simulink model "asbdhc2"  (Simulink 8.0)
settings: Solver=ode45  StartTime=0.0  StopTime=1000  MaxStep=1/30  RelTol=1e-2  AbsTol=1e-3
PreLoadFcn:
  | load asbdhc2_init;
values from neighbouring files (symbols this model uses):
  beaver_b = 14.63    [beaver_4_14_2013.mat]    (also in modelScript.m = 1.4224; monteCarloSim01.mat = 1.4224; simData_12_10_2013.mat = 1.4224; simData_12_9_2013.mat = 1.4224)
  beaver_c = 1.5875    [beaver_4_14_2013.mat]    (also in modelScript.m = 0.3302; monteCarloSim01.mat = 0.3302; simData_12_10_2013.mat = 0.3302; simData_12_9_2013.mat = 0.3302)
  beaver_init_p = 0    [beaver_4_14_2013.mat]    (also in monteCarloSim01.mat; simData_12_10_2013.mat; simData_12_9_2013.mat; simData_4_23_2013.mat)
  beaver_init_pitch = 0.13029612885    [beaver_4_14_2013.mat]    (also in monteCarloSim01.mat; simData_12_10_2013.mat; simData_12_9_2013.mat; simData_4_23_2013.mat)
  beaver_init_q = 0    [beaver_4_14_2013.mat]    (also in monteCarloSim01.mat; simData_12_10_2013.mat; simData_12_9_2013.mat; simData_4_23_2013.mat)
  beaver_init_r = 0    [beaver_4_14_2013.mat]    (also in monteCarloSim01.mat; simData_12_10_2013.mat; simData_12_9_2013.mat; simData_4_23_2013.mat)
  beaver_init_roll = 0    [beaver_4_14_2013.mat]    (also in monteCarloSim01.mat; simData_12_10_2013.mat; simData_12_9_2013.mat; simData_4_23_2013.mat)
  beaver_mass = 2288.231    [beaver_4_14_2013.mat]    (also in modelScript.m = 1.56; monteCarloSim01.mat = 1.56; simData_12_10_2013.mat = 1.56; simData_12_9_2013.mat = 1.56)
  beaver_S = 23.23    [beaver_4_14_2013.mat]    (also in modelScript.m = 0.2589; monteCarloSim01.mat = 0.2589; simData_12_10_2013.mat = 0.2589; simData_12_9_2013.mat = 0.2589)
  CD0 = 0.03    [modelScript.m]    (also in monteCarloSim01.mat; polarFun.m = x(1); simData_12_10_2013.mat; simData_12_9_2013.mat)
  Cl0 = 0.000591    [beaver_4_14_2013.mat]    (also in monteCarloSim01.mat; simData_12_10_2013.mat; simData_12_9_2013.mat; simData_4_23_2013.mat)
  Cl_alpha2_dpt = -0.01406    [beaver_4_14_2013.mat]    (also in monteCarloSim01.mat; simData_12_10_2013.mat; simData_12_9_2013.mat; simData_4_23_2013.mat)
  Cl_beta = -0.0618    [beaver_4_14_2013.mat]    (also in monteCarloSim01.mat; simData_12_10_2013.mat; simData_12_9_2013.mat; simData_4_23_2013.mat)
  Cl_da = -0.09917    [beaver_4_14_2013.mat]    (also in monteCarloSim01.mat; simData_12_10_2013.mat; simData_12_9_2013.mat; simData_4_23_2013.mat)
  Cl_da_alpha = -0.08269    [beaver_4_14_2013.mat]    (also in monteCarloSim01.mat; simData_12_10_2013.mat; simData_12_9_2013.mat; simData_4_23_2013.mat)
  Cl_dr = 0.006934    [beaver_4_14_2013.mat]    (also in monteCarloSim01.mat; simData_12_10_2013.mat; simData_12_9_2013.mat; simData_4_23_2013.mat)
  Cl_p = -0.5045    [beaver_4_14_2013.mat]    (also in monteCarloSim01.mat; simData_12_10_2013.mat; simData_12_9_2013.mat; simData_4_23_2013.mat)
  Cl_r = 0.1695    [beaver_4_14_2013.mat]    (also in monteCarloSim01.mat; simData_12_10_2013.mat; simData_12_9_2013.mat; simData_4_23_2013.mat)
  Cm0 = 0.09448    [beaver_4_14_2013.mat]    (also in monteCarloSim01.mat; simData_12_10_2013.mat; simData_12_9_2013.mat; simData_4_23_2013.mat)
  Cm_alpha = -0.6028    [beaver_4_14_2013.mat]    (also in monteCarloSim01.mat; simData_12_10_2013.mat; simData_12_9_2013.mat; simData_4_23_2013.mat)
  Cm_alpha2 = -2.14    [beaver_4_14_2013.mat]    (also in monteCarloSim01.mat; simData_12_10_2013.mat; simData_12_9_2013.mat; simData_4_23_2013.mat)
  Cm_beta2 = 0.6921    [beaver_4_14_2013.mat]    (also in monteCarloSim01.mat; simData_12_10_2013.mat; simData_12_9_2013.mat; simData_4_23_2013.mat)
  Cm_de = -1.921    [beaver_4_14_2013.mat]    (also in monteCarloSim01.mat; simData_12_10_2013.mat; simData_12_9_2013.mat; simData_4_23_2013.mat)
  Cm_df = 0.4072    [beaver_4_14_2013.mat]    (also in monteCarloSim01.mat; simData_12_10_2013.mat; simData_12_9_2013.mat; simData_4_23_2013.mat)
  Cm_dpt = -0.07895    [beaver_4_14_2013.mat]    (also in monteCarloSim01.mat; simData_12_10_2013.mat; simData_12_9_2013.mat; simData_4_23_2013.mat)
  Cm_q = -15.56    [beaver_4_14_2013.mat]    (also in monteCarloSim01.mat; simData_12_10_2013.mat; simData_12_9_2013.mat; simData_4_23_2013.mat)
  Cm_r = -0.3118    [beaver_4_14_2013.mat]    (also in monteCarloSim01.mat; simData_12_10_2013.mat; simData_12_9_2013.mat; simData_4_23_2013.mat)
  Cn0 = -0.003117    [beaver_4_14_2013.mat]    (also in monteCarloSim01.mat; simData_12_10_2013.mat; simData_12_9_2013.mat; simData_4_23_2013.mat)
  Cn_beta = 0.006719    [beaver_4_14_2013.mat]    (also in monteCarloSim01.mat; simData_12_10_2013.mat; simData_12_9_2013.mat; simData_4_23_2013.mat)
  Cn_beta3 = 0.1373    [beaver_4_14_2013.mat]    (also in monteCarloSim01.mat; simData_12_10_2013.mat; simData_12_9_2013.mat; simData_4_23_2013.mat)
  Cn_da = -0.003872    [beaver_4_14_2013.mat]    (also in monteCarloSim01.mat; simData_12_10_2013.mat; simData_12_9_2013.mat; simData_4_23_2013.mat)
  Cn_dpt3 = -0.003026    [beaver_4_14_2013.mat]    (also in monteCarloSim01.mat; simData_12_10_2013.mat; simData_12_9_2013.mat; simData_4_23_2013.mat)
  Cn_dr = -0.08265    [beaver_4_14_2013.mat]    (also in monteCarloSim01.mat; simData_12_10_2013.mat; simData_12_9_2013.mat; simData_4_23_2013.mat)
  Cn_p = -0.1585    [beaver_4_14_2013.mat]    (also in monteCarloSim01.mat; simData_12_10_2013.mat; simData_12_9_2013.mat; simData_4_23_2013.mat)
  Cn_q = 0.1595    [beaver_4_14_2013.mat]    (also in monteCarloSim01.mat; simData_12_10_2013.mat; simData_12_9_2013.mat; simData_4_23_2013.mat)
  Cn_r = -0.1112    [beaver_4_14_2013.mat]    (also in monteCarloSim01.mat; simData_12_10_2013.mat; simData_12_9_2013.mat; simData_4_23_2013.mat)
  Cx0 = -0.03554    [beaver_4_14_2013.mat]    (also in modelScript.m = 0; monteCarloSim01.mat = 0; simData_12_10_2013.mat = 0; simData_12_9_2013.mat = 0)
  Cx_alpha = 0.00292    [beaver_4_14_2013.mat]    (also in modelScript.m = 0; monteCarloSim01.mat = 0; simData_12_10_2013.mat = 0; simData_12_9_2013.mat = 0)
  Cx_alpha2 = 5.459    [beaver_4_14_2013.mat]    (also in modelScript.m = 0; monteCarloSim01.mat = 0; simData_12_10_2013.mat = 0; simData_12_9_2013.mat = 0)
  Cx_alpha3 = -5.162    [beaver_4_14_2013.mat]    (also in modelScript.m = 0; monteCarloSim01.mat = 0; simData_12_10_2013.mat = 0; simData_12_9_2013.mat = 0)
  Cx_df = -0.09447    [beaver_4_14_2013.mat]    (also in modelScript.m = 0; monteCarloSim01.mat = 0; simData_12_10_2013.mat = 0; simData_12_9_2013.mat = 0)
  Cx_df_alpha = 1.106    [beaver_4_14_2013.mat]    (also in modelScript.m = 0; monteCarloSim01.mat = 0; simData_12_10_2013.mat = 0; simData_12_9_2013.mat = 0)
  Cx_dpt = 0.1161    [beaver_4_14_2013.mat]    (also in modelScript.m = 0; monteCarloSim01.mat = 0; simData_12_10_2013.mat = 0; simData_12_9_2013.mat = 0)
  Cx_dpt2_alpha = 0.1453    [beaver_4_14_2013.mat]    (also in modelScript.m = 0; monteCarloSim01.mat = 0; simData_12_10_2013.mat = 0; simData_12_9_2013.mat = 0)
  Cx_dr = 0.03412    [beaver_4_14_2013.mat]    (also in modelScript.m = 0; monteCarloSim01.mat = 0; simData_12_10_2013.mat = 0; simData_12_9_2013.mat = 0)
  Cx_q = -0.6748    [beaver_4_14_2013.mat]    (also in modelScript.m = 0; monteCarloSim01.mat = 0; simData_12_10_2013.mat = 0; simData_12_9_2013.mat = 0)
  Cy0 = -0.002226    [beaver_4_14_2013.mat]    (also in modelScript.m = 0; monteCarloSim01.mat = 0; simData_12_10_2013.mat = 0; simData_12_9_2013.mat = 0)
  Cy_beta = -0.7678    [beaver_4_14_2013.mat]    (also in modelScript.m = 0; monteCarloSim01.mat = 0; simData_12_10_2013.mat = 0; simData_12_9_2013.mat = 0)
  Cy_da = -0.02956    [beaver_4_14_2013.mat]    (also in modelScript.m = 0; monteCarloSim01.mat = 0; simData_12_10_2013.mat = 0; simData_12_9_2013.mat = 0)
  Cy_dr = 0.1158    [beaver_4_14_2013.mat]    (also in modelScript.m = 0; monteCarloSim01.mat = 0; simData_12_10_2013.mat = 0; simData_12_9_2013.mat = 0)
  Cy_dr_alpha = 0.5238    [beaver_4_14_2013.mat]    (also in modelScript.m = 0; monteCarloSim01.mat = 0; simData_12_10_2013.mat = 0; simData_12_9_2013.mat = 0)
  Cy_p = -0.124    [beaver_4_14_2013.mat]    (also in modelScript.m = 0; monteCarloSim01.mat = 0; simData_12_10_2013.mat = 0; simData_12_9_2013.mat = 0)
  Cy_r = 0.3666    [beaver_4_14_2013.mat]    (also in modelScript.m = 0; monteCarloSim01.mat = 0; simData_12_10_2013.mat = 0; simData_12_9_2013.mat = 0)
  Cz0 = -0.05504    [beaver_4_14_2013.mat]    (also in modelScript.m = 0; monteCarloSim01.mat = 0; simData_12_10_2013.mat = 0; simData_12_9_2013.mat = 0)
  Cz_alpha = -5.578    [beaver_4_14_2013.mat]    (also in modelScript.m = 0; monteCarloSim01.mat = 0; simData_12_10_2013.mat = 0; simData_12_9_2013.mat = 0)
  Cz_alpha3 = 3.442    [beaver_4_14_2013.mat]    (also in modelScript.m = 0; monteCarloSim01.mat = 0; simData_12_10_2013.mat = 0; simData_12_9_2013.mat = 0)
  Cz_de = -0.398    [beaver_4_14_2013.mat]    (also in modelScript.m = 0; monteCarloSim01.mat = 0; simData_12_10_2013.mat = 0; simData_12_9_2013.mat = 0)
  Cz_de_beta = -15.93    [beaver_4_14_2013.mat]    (also in modelScript.m = 0; monteCarloSim01.mat = 0; simData_12_10_2013.mat = 0; simData_12_9_2013.mat = 0)
  Cz_df = -1.377    [beaver_4_14_2013.mat]    (also in modelScript.m = 0; monteCarloSim01.mat = 0; simData_12_10_2013.mat = 0; simData_12_9_2013.mat = 0)
  Cz_df_alpha = -1.261    [beaver_4_14_2013.mat]    (also in modelScript.m = 0; monteCarloSim01.mat = 0; simData_12_10_2013.mat = 0; simData_12_9_2013.mat = 0)
  Cz_dpt = -0.1563    [beaver_4_14_2013.mat]    (also in modelScript.m = 0; monteCarloSim01.mat = 0; simData_12_10_2013.mat = 0; simData_12_9_2013.mat = 0)
  Cz_q = -2.988    [beaver_4_14_2013.mat]    (also in modelScript.m = 0; monteCarloSim01.mat = 0; simData_12_10_2013.mat = 0; simData_12_9_2013.mat = 0)
  Ix = .1147    (= 0.1147)    [modelScript.m]    (also in monteCarloSim01.mat; simData_12_10_2013.mat; simData_12_9_2013.mat; simData_4_26_2013.mat)
  Ixz = .0015    (= 0.0015)    [modelScript.m]    (also in monteCarloSim01.mat; simData_12_10_2013.mat; simData_12_9_2013.mat; simData_4_26_2013.mat)
  Iy = .0576    (= 0.0576)    [modelScript.m]    (also in monteCarloSim01.mat; simData_12_10_2013.mat; simData_12_9_2013.mat; simData_4_26_2013.mat)
  Iz = .1712    (= 0.1712)    [modelScript.m]    (also in monteCarloSim01.mat; simData_12_10_2013.mat; simData_12_9_2013.mat; simData_4_26_2013.mat)
  KCL2 = 1/(pi*.7*beaver_b/beaver_c)    [modelScript.m]    (also in monteCarloSim01.mat = 0.0493425392361; polarFun.m = x(2); simData_12_10_2013.mat = 0.0493425392361; simData_12_9_2013.mat = 0.0493425392361)
  m = state.W/g(1)    [plant.m]
  nonLinearCd = [0.025 0.0283582705905 0.0317165411809 0.0350748117714 0.0384330823618 0.0417913529523 0.0451496235427 0.0485078941332 0.0518661647236 0.0552244353141 0.0585827059046 0.061940976495 ... (1000 elements, 1x1000)]    [NACA0012Adam.mat]    (also in monteCarloSim01.mat; simData_12_10_2013.mat; simData_12_9_2013.mat; simData_4_23_2013.mat)
  nonLinearCl = [0 0.0485067508622 0.0970135017244 0.145520252587 0.194027003449 0.240505289572 0.286480266666 0.332455243759 0.378430220853 0.421875006681 0.463843622747 0.505812238814 ... (1000 elements, 1x1000)]    [NACA0012Adam.mat]    (also in monteCarloSim01.mat; simData_12_10_2013.mat; simData_12_9_2013.mat; simData_4_23_2013.mat)
  nonLinearWindAeroAlpha = [-3.14159265359 -3.13530317881 -3.12901370403 -3.12272422924 -3.11643475446 -3.11014527968 -3.1038558049 -3.09756633012 -3.09127685533 -3.08498738055 -3.07869790577 -3.07240843099 ... (1000 elements, 1x1000)]    [NACA0012Adam.mat]    (also in monteCarloSim01.mat; simData_12_10_2013.mat; simData_12_9_2013.mat; simData_4_23_2013.mat)
  q = state.eulerRates(:,2)    [eulerKalman.m]
  r = state.eulerRates(:,3)    [eulerKalman.m]
  sampleVec = [1/1000 0]    [modelScript.m]    (also in monteCarloSim01.mat = [0.0909090909091 0]; simData_12_10_2013.mat = [0.0909090909091 0]; simData_12_9_2013.mat = [0.001 0]; simData_4_26_2013.mat = [0.02 0])
  u0 = 100/3.28    (= 30.487804878)    [modelScript.m]    (also in monteCarloSim01.mat; simData_12_10_2013.mat; simData_12_9_2013.mat; simData_4_26_2013.mat)
  uaero0 = [-0.0317656979071 -0.0320210159663 -0.0365180369264 0]    [beaver_4_14_2013.mat]    (also in monteCarloSim01.mat; simData_12_10_2013.mat; simData_12_9_2013.mat; simData_4_23_2013.mat)
  v0 = 0    [modelScript.m]    (also in monteCarloSim01.mat; simData_12_10_2013.mat; simData_12_9_2013.mat; simData_4_26_2013.mat)
  w0 = 0    [modelScript.m]    (also in monteCarloSim01.mat; simData_12_10_2013.mat; simData_12_9_2013.mat; simData_4_26_2013.mat)
undefined symbols (not defined in the file or in its folder): Earth, F, Light, MIL, s, sigbuilder_block, WGS84
libraries: aerolibconvert2 x5, aerolibtransform2 x4, aerolibadynsys x3, aerolibasang x3, aerolibwind2 x3, aerolibfltsims x3, aerolibanimutils x2, aerolib6dof2 x1, aerolibnav x1, aerolibutil x1, aerolibatmos2 x1, aerolibgravity2 x1
(part 2 of 2)

== system asbdhc2/DeHavilland Beaver Airframe/Aircraft Dynamics/Total Forces  and Moments/Aerodynamics/Body Rate Damping ==
  V : Inport
  p,q,r : Inport  Port=2
  Demux : Demux  Outputs=3
  Product : Product  SaturateOnIntegerOverflow=on  InputSameDT=on  OutDataTypeStr=Inherit: Same as first input
  Product1 : Product  SaturateOnIntegerOverflow=on  InputSameDT=on  OutDataTypeStr=Inherit: Same as first input
  Product2 : Product  SaturateOnIntegerOverflow=on  InputSameDT=on  OutDataTypeStr=Inherit: Same as first input
  Product3 : Product  Inputs=*/  SaturateOnIntegerOverflow=on  InputSameDT=on  OutDataTypeStr=Inherit: Same as first input
  Reference Length : Gain  Gain=beaver_c  SaturateOnIntegerOverflow=on  OutDataTypeStr=Inherit: Same as input  ParamDataTypeStr=Inherit: Same as input
  Reference Span : Gain  Gain=beaver_b/2  SaturateOnIntegerOverflow=on  OutDataTypeStr=Inherit: Same as input  ParamDataTypeStr=Inherit: Same as input
  "Reference Span " : Gain  Gain=beaver_b/2  SaturateOnIntegerOverflow=on  OutDataTypeStr=Inherit: Same as input  ParamDataTypeStr=Inherit: Same as input
  Sum1 : Sum  Inputs=+++  SaturateOnIntegerOverflow=on  InputSameDT=on  OutDataTypeStr=Inherit: Same as first input
  p : Subsystem
  q : Subsystem
  r : Subsystem
  Coefficients : Outport
  wires:
  p/1(delCoeff) -> Product/1
  q/1(delCoeff) -> Product1/1
  p,q,r/1 -> Demux/1
  Demux/1 -> Product/2  "p"
  Demux/2 -> Product1/2  "q"
  Demux/3 -> Product2/2  "r"
  Sum1/1 -> Product3/1
  V/1 -> Product3/2
  Product3/1 -> Coefficients/1
  Product1/1 -> Reference Length/1
  Product2/1 -> "Reference Span "/1
  Product/1 -> Reference Span/1
  r/1(delCoeff) -> Product2/1
  Reference Length/1 -> Sum1/2
  Reference Span/1 -> Sum1/1
  "Reference Span "/1 -> Sum1/3

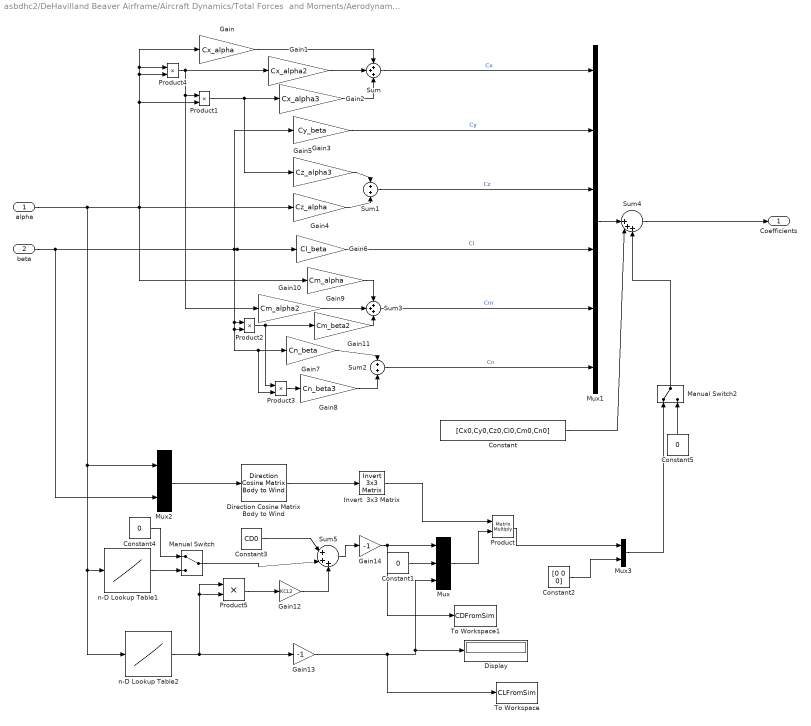
== system asbdhc2/DeHavilland Beaver Airframe/Aircraft Dynamics/Total Forces  and Moments/Aerodynamics/Datum Coefficients ==
  alpha : Inport
  beta : Inport  Port=2
  Constant : Constant  Value=[Cx0,Cy0,Cz0,Cl0,Cm0,Cn0]
  Constant1 : Constant  Value=0
  Constant2 : Constant  Value=[0 0 0]
  Constant3 : Constant  Value=CD0
  Constant4 : Constant  Value=0
  Constant5 : Constant  Value=0
  Direction Cosine Matrix Body to Wind : aerolibtransform2/Direction Cosine Matrix Body to Wind
  Display : Display
  Gain : Gain  Gain=Cx_alpha  SaturateOnIntegerOverflow=on  OutDataTypeStr=Inherit: Same as input  ParamDataTypeStr=Inherit: Same as input
  Gain1 : Gain  Gain=Cx_alpha2  SaturateOnIntegerOverflow=on  OutDataTypeStr=Inherit: Same as input  ParamDataTypeStr=Inherit: Same as input
  Gain10 : Gain  Gain=Cm_alpha2  SaturateOnIntegerOverflow=on  OutDataTypeStr=Inherit: Same as input  ParamDataTypeStr=Inherit: Same as input
  Gain11 : Gain  Gain=Cm_beta2  SaturateOnIntegerOverflow=on  OutDataTypeStr=Inherit: Same as input  ParamDataTypeStr=Inherit: Same as input
  Gain12 : Gain  Gain=KCL2
  Gain13 : Gain  Gain=-1
  Gain14 : Gain  Gain=-1
  Gain2 : Gain  Gain=Cx_alpha3  SaturateOnIntegerOverflow=on  OutDataTypeStr=Inherit: Same as input  ParamDataTypeStr=Inherit: Same as input
  Gain3 : Gain  Gain=Cy_beta  SaturateOnIntegerOverflow=on  OutDataTypeStr=Inherit: Same as input  ParamDataTypeStr=Inherit: Same as input
  Gain4 : Gain  Gain=Cz_alpha  SaturateOnIntegerOverflow=on  OutDataTypeStr=Inherit: Same as input  ParamDataTypeStr=Inherit: Same as input
  Gain5 : Gain  Gain=Cz_alpha3  SaturateOnIntegerOverflow=on  OutDataTypeStr=Inherit: Same as input  ParamDataTypeStr=Inherit: Same as input
  Gain6 : Gain  Gain=Cl_beta  SaturateOnIntegerOverflow=on  OutDataTypeStr=Inherit: Same as input  ParamDataTypeStr=Inherit: Same as input
  Gain7 : Gain  Gain=Cn_beta  SaturateOnIntegerOverflow=on  OutDataTypeStr=Inherit: Same as input  ParamDataTypeStr=Inherit: Same as input
  Gain8 : Gain  Gain=Cn_beta3  SaturateOnIntegerOverflow=on  OutDataTypeStr=Inherit: Same as input  ParamDataTypeStr=Inherit: Same as input
  Gain9 : Gain  Gain=Cm_alpha  SaturateOnIntegerOverflow=on  OutDataTypeStr=Inherit: Same as input  ParamDataTypeStr=Inherit: Same as input
  Invert  3x3 Matrix : aerolibutil/Invert  3x3 Matrix
  Manual Switch : ManualSwitch
  Manual Switch2 : ManualSwitch
  Mux : Mux  Inputs=3
  Mux1 : Mux  Inputs=6
  Mux2 : Mux  Inputs=2
  Mux3 : Mux  Inputs=[3 3]
  Product : Product  Multiplication=Matrix(*)  RndMeth=Zero
  Product{1..4} (4 alike) : Product  SaturateOnIntegerOverflow=on  InputSameDT=on  OutDataTypeStr=Inherit: Same as first input
  Product5 : Product  RndMeth=Zero
  Sum : Sum  Inputs=+++  SaturateOnIntegerOverflow=on
  Sum1 : Sum  SaturateOnIntegerOverflow=on
  Sum2 : Sum  SaturateOnIntegerOverflow=on
  Sum3 : Sum  Inputs=+++  SaturateOnIntegerOverflow=on
  Sum4 : Sum  Inputs=||+++  SaturateOnIntegerOverflow=on
  Sum5 : Sum  Inputs=|+++  SaturateOnIntegerOverflow=on
  To Workspace : ToWorkspace  VariableName=CLFromSim  SampleTime=-1  SaveFormat=Structure
  To Workspace1 : ToWorkspace  VariableName=CDFromSim  SampleTime=-1  SaveFormat=Structure
  n-D Lookup Table1 : Lookup_n-D  NumberOfTableDimensions=1  BreakpointsForDimension1=nonLinearWindAeroAlpha  Table=nonLinearCd  RndMeth=Simplest  InputSameDT=on
  n-D Lookup Table2 : Lookup_n-D  NumberOfTableDimensions=1  BreakpointsForDimension1=nonLinearWindAeroAlpha  Table=nonLinearCl  RndMeth=Simplest  InputSameDT=on
  Coefficients : Outport
  wires:
  Constant/1 -> Sum4/2
  Sum4/1 -> Coefficients/1
  Mux1/1 -> Sum4/1
  Gain10/1 -> Sum3/2
  Product2/1 -> Product3/1, Gain11/1
  Gain11/1 -> Sum3/3
  Gain9/1 -> Sum3/1
  Sum3/1 -> Mux1/5  "Cm"
  Product3/1 -> Gain8/1
  Gain8/1 -> Sum2/2
  Gain7/1 -> Sum2/1
  Gain5/1 -> Sum1/1
  Gain4/1 -> Sum1/2
  Product1/1 -> Gain5/1, Gain2/1
  Gain2/1 -> Sum/3
  Product4/1 -> Product1/1, Gain10/1, Gain1/1
  Gain1/1 -> Sum/2
  Gain/1 -> Sum/1
  Sum2/1 -> Mux1/6  "Cn"
  Sum/1 -> Mux1/1  "Cx"
  Sum1/1 -> Mux1/3  "Cz"
  Gain3/1 -> Mux1/2  "Cy"
  Gain6/1 -> Mux1/4  "Cl"
  alpha/1 -> Product1/2, Product4/2, Product4/1, Gain/1, Gain9/1, Gain4/1, Mux2/1, n-D Lookup Table2/1, n-D Lookup Table1/1
  beta/1 -> Gain3/1, Product3/2, Gain7/1, Product2/2, Product2/1, Gain6/1, Mux2/2
  Mux2/1 -> Direction Cosine Matrix Body to Wind/1
  Direction Cosine Matrix Body to Wind/1 -> Invert  3x3 Matrix/1
  Invert  3x3 Matrix/1 -> Product/1
  Constant1/1 -> Mux/2
  Gain13/1 -> Mux/3, Display/1, To Workspace/1
  Constant2/1 -> Mux3/2
  Product/1 -> Mux3/1
  n-D Lookup Table2/1 -> Product5/2, Product5/1, Gain13/1
  Mux/1 -> Product/2
  Product5/1 -> Gain12/1
  Constant3/1 -> Sum5/1
  Gain14/1 -> Mux/1, To Workspace1/1
  Sum5/1 -> Gain14/1
  Gain12/1 -> Sum5/3
  n-D Lookup Table1/1 -> Manual Switch/2
  Constant4/1 -> Manual Switch/1
  Manual Switch/1 -> Sum5/2
  Mux3/1 -> Manual Switch2/1
  Manual Switch2/1 -> Sum4/3
  Constant5/1 -> Manual Switch2/2

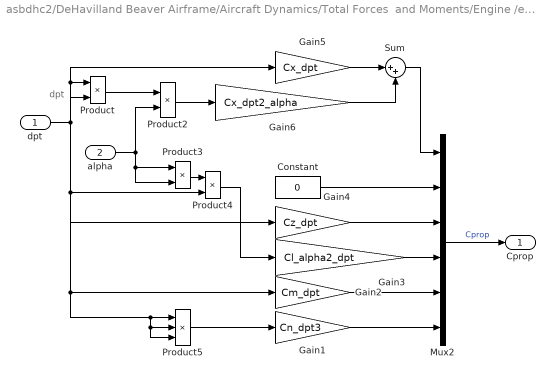
== system asbdhc2/DeHavilland Beaver Airframe/Aircraft Dynamics/Total Forces  and Moments/Engine /eng ==
  note: dpt
  dpt : Inport
  alpha : Inport  Port=2
  Constant : Constant  Value=0
  Gain1 : Gain  Gain=Cn_dpt3  SaturateOnIntegerOverflow=on  OutDataTypeStr=Inherit: Same as input  ParamDataTypeStr=Inherit: Same as input
  Gain2 : Gain  Gain=Cm_dpt  SaturateOnIntegerOverflow=on  OutDataTypeStr=Inherit: Same as input  ParamDataTypeStr=Inherit: Same as input
  Gain3 : Gain  Gain=Cl_alpha2_dpt  SaturateOnIntegerOverflow=on  OutDataTypeStr=Inherit: Same as input  ParamDataTypeStr=Inherit: Same as input
  Gain4 : Gain  Gain=Cz_dpt  SaturateOnIntegerOverflow=on  OutDataTypeStr=Inherit: Same as input  ParamDataTypeStr=Inherit: Same as input
  Gain5 : Gain  Gain=Cx_dpt  SaturateOnIntegerOverflow=on  OutDataTypeStr=Inherit: Same as input  ParamDataTypeStr=Inherit: Same as input
  Gain6 : Gain  Gain=Cx_dpt2_alpha  SaturateOnIntegerOverflow=on  OutDataTypeStr=Inherit: Same as input  ParamDataTypeStr=Inherit: Same as input
  Mux2 : Mux  Inputs=6
  Product{,2..4} (4 alike) : Product  SaturateOnIntegerOverflow=on  OutDataTypeStr=Inherit: Same as first input
  Product5 : Product  Inputs=3  SaturateOnIntegerOverflow=on  OutDataTypeStr=Inherit: Same as first input
  Sum : Sum  Inputs=|++  SaturateOnIntegerOverflow=on
  Cprop : Outport
  wires:
  Product5/1 -> Gain1/1
  Sum/1 -> Mux2/1
  Gain6/1 -> Sum/2
  Gain5/1 -> Sum/1
  Constant/1 -> Mux2/2
  Gain4/1 -> Mux2/3
  Gain3/1 -> Mux2/4
  Gain2/1 -> Mux2/5
  Gain1/1 -> Mux2/6
  Product4/1 -> Gain3/1
  Product2/1 -> Gain6/1
  dpt/1 -> Gain5/1, Product5/3, Product5/2, Product5/1, Gain2/1, Gain4/1, Product/2, Product/1, Product4/2
  alpha/1 -> Product2/2, Product3/1, Product3/2
  Mux2/1 -> Cprop/1  "Cprop"
  Product/1 -> Product2/1
  Product3/1 -> Product4/1

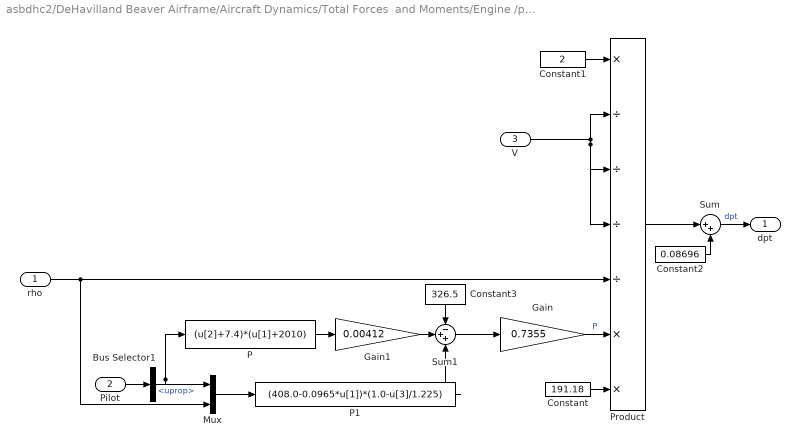
== system asbdhc2/DeHavilland Beaver Airframe/Aircraft Dynamics/Total Forces  and Moments/Engine /pow ==
  rho : Inport
  Pilot : Inport  Port=2
  V : Inport  Port=3
  Bus Selector1 : BusSelector  OutputSignals=uprop
  Constant : Constant  Value=191.18
  Constant1 : Constant  Value=2
  Constant2 : Constant  Value=0.08696
  Constant3 : Constant  Value=326.5
  Gain : Gain  Gain=0.7355  SaturateOnIntegerOverflow=on  OutDataTypeStr=Inherit: Same as input  ParamDataTypeStr=Inherit: Same as input
  Gain1 : Gain  Gain=0.00412  SaturateOnIntegerOverflow=on  OutDataTypeStr=Inherit: Same as input  ParamDataTypeStr=Inherit: Same as input
  Mux : Mux  Inputs=2
  P : Fcn  Expr=(u[2]+7.4)*(u[1]+2010)
  P1 : Fcn  Expr=(408.0-0.0965*u[1])*(1.0-u[3]/1.225)
  Product : Product  Inputs=*////**  SaturateOnIntegerOverflow=on  OutDataTypeStr=Inherit: Same as first input
  Sum : Sum  Inputs=|++  SaturateOnIntegerOverflow=on
  Sum1 : Sum  Inputs=-++  SaturateOnIntegerOverflow=on
  dpt : Outport
  wires:
  P1/1 -> Sum1/3
  Constant3/1 -> Sum1/1
  Gain1/1 -> Sum1/2
  Mux/1 -> P1/1
  Sum1/1 -> Gain/1
  P/1 -> Gain1/1
  Gain/1 -> Product/6  "P"
  rho/1 -> Mux/2, Product/5
  Sum/1 -> dpt/1  "dpt"
  V/1 -> Product/4, Product/3, Product/2
  Bus Selector1/1 -> P/1, Mux/1  "<uprop>"
  Constant/1 -> Product/7
  Constant1/1 -> Product/1
  Product/1 -> Sum/1
  Constant2/1 -> Sum/2
  Pilot/1 -> Bus Selector1/1

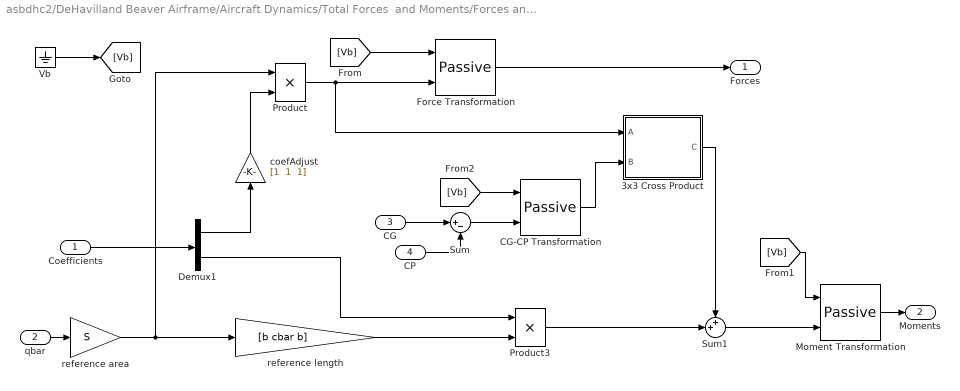
== system asbdhc2/DeHavilland Beaver Airframe/Aircraft Dynamics/Total Forces  and Moments/Forces and Moments/Aerodynamic Forces and Moments ==
  Coefficients : Inport
  qbar : Inport  Port=2
  CG : Inport  Port=3
  CP : Inport  Port=4
  3x3 Cross Product : Subsystem  AncestorBlock=aerolibutil/3x3 Cross Product  mask(CrossProduct){}
      mask help: Calculate the cross product of two 3-by-1 vectors.
      mask init:
      | aeroicon('aeroblk');
      mask Help: eval('asbhelp(''threebythree_cross_product'')');
      mask Display:
      | text(.5,.5,'Cross\nProduct\nC = AxB', ...
      | 	'HorizontalAlignment','Center',...
      | 	'VerticalAlignment','middle')
  CG-CP Transformation : aerolibadynsys/Passive  SystemSampleTime=-1
  Demux1 : Demux  Outputs=[3,3]
  Force Transformation : aerolibadynsys/Passive  SystemSampleTime=-1
  Moment Transformation : aerolibadynsys/Passive  SystemSampleTime=-1
  Product : Product  SaturateOnIntegerOverflow=on  InputSameDT=on  OutDataTypeStr=Inherit: Same as first input
  Product3 : Product  SaturateOnIntegerOverflow=on  InputSameDT=on  OutDataTypeStr=Inherit: Same as first input
  Sum : Sum  Inputs=|+-  SaturateOnIntegerOverflow=on
  Sum1 : Sum  Inputs=++|  SaturateOnIntegerOverflow=on  InputSameDT=on  OutDataTypeStr=Inherit: Same as first input
  Vb : Ground
  coefAdjust : Gain  Gain="[1  1  1]"
  reference area : Gain  Gain=S  SaturateOnIntegerOverflow=on  OutDataTypeStr=Inherit: Same as input  ParamDataTypeStr=Inherit: Same as input
  reference length : Gain  Gain=[b cbar b]  SaturateOnIntegerOverflow=on  OutDataTypeStr=Inherit: Same as input  ParamDataTypeStr=Inherit: Same as input
  Forces : Outport
  Moments : Outport  Port=2
  wires:
  3x3 Cross Product/1(C) -> Sum1/1
  reference length/1 -> Product3/2
  Coefficients/1 -> Demux1/1
  Demux1/2 -> Product3/1
  qbar/1 -> reference area/1
  reference area/1 -> Product/1, reference length/1
  Product3/1 -> Sum1/2
  Demux1/1 -> coefAdjust/1
  Product/1 -> Force Transformation/2, 3x3 Cross Product/1(A)
  Force Transformation/1 -> Forces/1
  Vb/1 -> [Vb]
  [Vb] -> Force Transformation/1
  Sum1/1 -> Moment Transformation/2
  Moment Transformation/1 -> Moments/1
  [Vb] -> Moment Transformation/1
  coefAdjust/1 -> Product/2
  CG/1 -> Sum/1
  CP/1 -> Sum/2
  Sum/1 -> CG-CP Transformation/2
  CG-CP Transformation/1 -> 3x3 Cross Product/2(B)
  [Vb] -> CG-CP Transformation/1

== system asbdhc2/DeHavilland Beaver Airframe/Aircraft Dynamics/Total Forces  and Moments/Aerodynamics/Actuator Increments/Aileron ==
  alpha : Inport
  Actuators : Inport  Port=2
  Gain1 : Gain  Gain=0  SaturateOnIntegerOverflow=on  OutDataTypeStr=Inherit: Same as input  ParamDataTypeStr=Inherit: Same as input
  Gain2 : Gain  Gain=Cy_da  SaturateOnIntegerOverflow=on  OutDataTypeStr=Inherit: Same as input  ParamDataTypeStr=Inherit: Same as input
  Gain3 : Gain  Gain=0  SaturateOnIntegerOverflow=on  OutDataTypeStr=Inherit: Same as input  ParamDataTypeStr=Inherit: Same as input
  Gain4 : Gain  Gain=Cn_da  SaturateOnIntegerOverflow=on  OutDataTypeStr=Inherit: Same as input  ParamDataTypeStr=Inherit: Same as input
  Gain5 : Gain  Gain=0  SaturateOnIntegerOverflow=on  OutDataTypeStr=Inherit: Same as input  ParamDataTypeStr=Inherit: Same as input
  Gain6 : Gain  Gain=Cl_da  SaturateOnIntegerOverflow=on  OutDataTypeStr=Inherit: Same as input  ParamDataTypeStr=Inherit: Same as input
  Gain7 : Gain  Gain=Cl_da_alpha  SaturateOnIntegerOverflow=on  OutDataTypeStr=Inherit: Same as input  ParamDataTypeStr=Inherit: Same as input
  Mux1 : Mux  Inputs=6
  Product4 : Product  SaturateOnIntegerOverflow=on  InputSameDT=on  OutDataTypeStr=Inherit: Same as first input
  Selector1 : Selector  InputPortWidth=4  IndexOptions=Index vector (dialog)  Indices=2  OutputSizes=1
  Sum1 : Sum  Inputs=++|  SaturateOnIntegerOverflow=on
  delCoeff : Outport
  wires:
  Gain6/1 -> Sum1/1
  Sum1/1 -> Mux1/4
  Gain7/1 -> Sum1/2
  Product4/1 -> Gain7/1
  Gain1/1 -> Mux1/1  "Cx"
  alpha/1 -> Product4/2
  Actuators/1 -> Selector1/1
  Mux1/1 -> delCoeff/1
  Gain2/1 -> Mux1/2  "Cy"
  Gain3/1 -> Mux1/3  "Cz"
  Gain5/1 -> Mux1/5  "Cm"
  Gain4/1 -> Mux1/6
  Selector1/1 -> Gain1/1, Gain2/1, Gain3/1, Gain6/1, Product4/1, Gain5/1, Gain4/1

== system asbdhc2/DeHavilland Beaver Airframe/Aircraft Dynamics/Total Forces  and Moments/Aerodynamics/Actuator Increments/Elevator ==
  Actuators : Inport
  Beta : Inport  Port=2
  Constant1 : Constant  Value=0
  Gain1 : Gain  Gain=Cz_de  SaturateOnIntegerOverflow=on  OutDataTypeStr=Inherit: Same as input  ParamDataTypeStr=Inherit: Same as input
  Gain2 : Gain  Gain=Cz_de_beta  SaturateOnIntegerOverflow=on  OutDataTypeStr=Inherit: Same as input  ParamDataTypeStr=Inherit: Same as input
  Gain3 : Gain  Gain=Cm_de  SaturateOnIntegerOverflow=on  OutDataTypeStr=Inherit: Same as input  ParamDataTypeStr=Inherit: Same as input
  Mux1 : Mux  Inputs=6
  Product4 : Product  Inputs=3  SaturateOnIntegerOverflow=on  InputSameDT=on  OutDataTypeStr=Inherit: Same as first input
  Selector1 : Selector  InputPortWidth=4  IndexOptions=Index vector (dialog)  Indices=1  OutputSizes=1
  Sum1 : Sum  SaturateOnIntegerOverflow=on
  delCoeff : Outport
  wires:
  Gain3/1 -> Mux1/5
  Gain1/1 -> Sum1/2
  Gain2/1 -> Sum1/1
  Sum1/1 -> Mux1/3
  Product4/1 -> Gain2/1
  Beta/1 -> Product4/2, Product4/1
  Mux1/1 -> delCoeff/1
  Selector1/1 -> Gain3/1, Gain1/1, Product4/3
  Constant1/1 -> Mux1/1, Mux1/2, Mux1/4, Mux1/6
  Actuators/1 -> Selector1/1

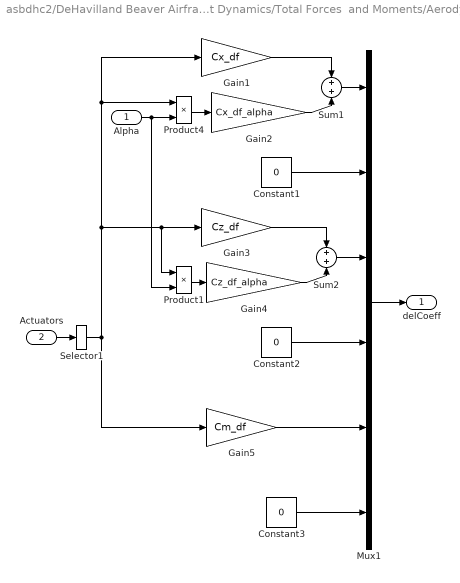
== system asbdhc2/DeHavilland Beaver Airframe/Aircraft Dynamics/Total Forces  and Moments/Aerodynamics/Actuator Increments/Flap ==
  Alpha : Inport
  Actuators : Inport  Port=2
  Constant1 : Constant  Value=0
  Constant2 : Constant  Value=0
  Constant3 : Constant  Value=0
  Gain1 : Gain  Gain=Cx_df  SaturateOnIntegerOverflow=on  OutDataTypeStr=Inherit: Same as input  ParamDataTypeStr=Inherit: Same as input
  Gain2 : Gain  Gain=Cx_df_alpha  SaturateOnIntegerOverflow=on  OutDataTypeStr=Inherit: Same as input  ParamDataTypeStr=Inherit: Same as input
  Gain3 : Gain  Gain=Cz_df  SaturateOnIntegerOverflow=on  OutDataTypeStr=Inherit: Same as input  ParamDataTypeStr=Inherit: Same as input
  Gain4 : Gain  Gain=Cz_df_alpha  SaturateOnIntegerOverflow=on  OutDataTypeStr=Inherit: Same as input  ParamDataTypeStr=Inherit: Same as input
  Gain5 : Gain  Gain=Cm_df  SaturateOnIntegerOverflow=on  OutDataTypeStr=Inherit: Same as input  ParamDataTypeStr=Inherit: Same as input
  Mux1 : Mux  Inputs=6
  Product1 : Product  SaturateOnIntegerOverflow=on  InputSameDT=on  OutDataTypeStr=Inherit: Same as first input
  Product4 : Product  SaturateOnIntegerOverflow=on  InputSameDT=on  OutDataTypeStr=Inherit: Same as first input
  Selector1 : Selector  InputPortWidth=4  IndexOptions=Index vector (dialog)  Indices=4  OutputSizes=1
  Sum1 : Sum  SaturateOnIntegerOverflow=on
  Sum2 : Sum  SaturateOnIntegerOverflow=on
  delCoeff : Outport
  wires:
  Selector1/1 -> Gain1/1, Product4/1, Product1/1, Gain3/1, Gain5/1
  Actuators/1 -> Selector1/1
  Gain5/1 -> Mux1/5
  Gain3/1 -> Sum2/1
  Gain4/1 -> Sum2/2
  Product1/1 -> Gain4/1
  Gain1/1 -> Sum1/1
  Gain2/1 -> Sum1/2
  Product4/1 -> Gain2/1
  Alpha/1 -> Product1/2, Product4/2
  Mux1/1 -> delCoeff/1
  Sum1/1 -> Mux1/1
  Sum2/1 -> Mux1/3
  Constant1/1 -> Mux1/2
  Constant2/1 -> Mux1/4
  Constant3/1 -> Mux1/6

== system asbdhc2/DeHavilland Beaver Airframe/Aircraft Dynamics/Total Forces  and Moments/Aerodynamics/Actuator Increments/Rudder ==
  Alpha : Inport
  Actuators : Inport  Port=2
  Constant1 : Constant  Value=0
  Constant2 : Constant  Value=0
  Gain1 : Gain  Gain=Cl_dr  SaturateOnIntegerOverflow=on  OutDataTypeStr=Inherit: Same as input  ParamDataTypeStr=Inherit: Same as input
  Gain2 : Gain  Gain=Cn_dr  SaturateOnIntegerOverflow=on  OutDataTypeStr=Inherit: Same as input  ParamDataTypeStr=Inherit: Same as input
  Gain3 : Gain  Gain=Cy_dr_alpha  SaturateOnIntegerOverflow=on  OutDataTypeStr=Inherit: Same as input  ParamDataTypeStr=Inherit: Same as input
  Gain4 : Gain  Gain=Cy_dr  SaturateOnIntegerOverflow=on  OutDataTypeStr=Inherit: Same as input  ParamDataTypeStr=Inherit: Same as input
  Gain5 : Gain  Gain=Cx_dr  SaturateOnIntegerOverflow=on  OutDataTypeStr=Inherit: Same as input  ParamDataTypeStr=Inherit: Same as input
  Mux1 : Mux  Inputs=6
  Product1 : Product  SaturateOnIntegerOverflow=on  InputSameDT=on  OutDataTypeStr=Inherit: Same as first input
  Selector1 : Selector  InputPortWidth=4  IndexOptions=Index vector (dialog)  Indices=3  OutputSizes=1
  Sum1 : Sum  SaturateOnIntegerOverflow=on
  delCoeff : Outport
  wires:
  Gain5/1 -> Mux1/1
  Gain4/1 -> Sum1/1
  Gain3/1 -> Sum1/2
  Gain1/1 -> Mux1/4
  Gain2/1 -> Mux1/6
  Product1/1 -> Gain3/1
  Alpha/1 -> Product1/2
  Mux1/1 -> delCoeff/1
  Actuators/1 -> Selector1/1
  Sum1/1 -> Mux1/2
  Constant1/1 -> Mux1/3
  Constant2/1 -> Mux1/5
  Selector1/1 -> Gain5/1, Gain4/1, Gain1/1, Gain2/1, Product1/1

== system asbdhc2/DeHavilland Beaver Airframe/Aircraft Dynamics/Total Forces  and Moments/Aerodynamics/Body Rate Damping/p ==
  Constant1 : Constant  Value=0
  Constant2 : Constant  Value=Cy_p
  Constant3 : Constant  Value=Cl_p
  Constant4 : Constant  Value=Cn_p
  Mux1 : Mux  Inputs=6
  delCoeff : Outport
  wires:
  Constant2/1 -> Mux1/2
  Mux1/1 -> delCoeff/1
  Constant1/1 -> Mux1/5, Mux1/3, Mux1/1
  Constant4/1 -> Mux1/6
  Constant3/1 -> Mux1/4

== system asbdhc2/DeHavilland Beaver Airframe/Aircraft Dynamics/Total Forces  and Moments/Aerodynamics/Body Rate Damping/q ==
  Constant1 : Constant  Value=0
  Constant2 : Constant  Value=Cz_q
  Constant3 : Constant  Value=Cx_q
  Constant4 : Constant  Value=Cm_q
  Constant5 : Constant  Value=Cn_q
  Mux1 : Mux  Inputs=6
  delCoeff : Outport
  wires:
  Constant2/1 -> Mux1/3
  Constant5/1 -> Mux1/6
  Constant1/1 -> Mux1/4, Mux1/2
  Constant4/1 -> Mux1/5
  Constant3/1 -> Mux1/1
  Mux1/1 -> delCoeff/1

== system asbdhc2/DeHavilland Beaver Airframe/Aircraft Dynamics/Total Forces  and Moments/Aerodynamics/Body Rate Damping/r ==
  Constant : Constant  Value=0
  Constant1 : Constant  Value=Cy_r
  Constant2 : Constant  Value=Cl_r
  Constant3 : Constant  Value=Cm_r
  Constant4 : Constant  Value=Cn_r
  Mux1 : Mux  Inputs=6
  delCoeff : Outport
  wires:
  Constant3/1 -> Mux1/5
  Constant1/1 -> Mux1/2
  Constant4/1 -> Mux1/6
  Constant2/1 -> Mux1/4
  Constant/1 -> Mux1/3, Mux1/1
  Mux1/1 -> delCoeff/1

== system asbdhc2/DeHavilland Beaver Airframe/Aircraft Dynamics/Total Forces  and Moments/Forces and Moments/Aerodynamic Forces and Moments/3x3 Cross Product ==
  A : Inport
  B : Inport  Port=2
  "A " : InportShadow
  "B " : InportShadow  Port=2
  Subsystem : Subsystem
  Subsystem1 : Subsystem
  Sum : Sum  Inputs=+|-  SaturateOnIntegerOverflow=on  InputSameDT=on  OutDataTypeStr=Inherit: Same as first input
  C : Outport
  wires:
  "B "/1 -> Subsystem1/2(B)
  "A "/1 -> Subsystem1/1(A)
  Sum/1 -> C/1
  B/1 -> Subsystem/2(B)
  A/1 -> Subsystem/1(A)
  Subsystem/1(Out1) -> Sum/1
  Subsystem1/1(Out1) -> Sum/2

== system asbdhc2/DeHavilland Beaver Airframe/Aircraft Dynamics/Total Forces  and Moments/Forces and Moments/Aerodynamic Forces and Moments/3x3 Cross Product/Subsystem ==
  A : Inport
  B : Inport  Port=2
  Demux : Demux  Outputs=3
  Demux1 : Demux  Outputs=3
  Mux : Mux  Inputs=3
  i x j : Product  SaturateOnIntegerOverflow=on  InputSameDT=on  OutDataTypeStr=Inherit: Same as first input
  j x k : Product  SaturateOnIntegerOverflow=on  InputSameDT=on  OutDataTypeStr=Inherit: Same as first input
  k x i : Product  SaturateOnIntegerOverflow=on  InputSameDT=on  OutDataTypeStr=Inherit: Same as first input
  Out1 : Outport
  wires:
  Demux1/3 -> j x k/2
  Demux/2 -> j x k/1
  Demux/3 -> k x i/1
  Demux1/1 -> k x i/2
  Demux1/2 -> i x j/2
  Demux/1 -> i x j/1
  i x j/1 -> Mux/3
  k x i/1 -> Mux/2
  j x k/1 -> Mux/1
  B/1 -> Demux1/1
  A/1 -> Demux/1
  Mux/1 -> Out1/1

== system asbdhc2/DeHavilland Beaver Airframe/Aircraft Dynamics/Total Forces  and Moments/Forces and Moments/Aerodynamic Forces and Moments/3x3 Cross Product/Subsystem1 ==
  A : Inport
  B : Inport  Port=2
  Demux : Demux  Outputs=3
  Demux1 : Demux  Outputs=3
  Mux : Mux  Inputs=3
  i x k : Product  SaturateOnIntegerOverflow=on  InputSameDT=on  OutDataTypeStr=Inherit: Same as first input
  j x i : Product  SaturateOnIntegerOverflow=on  InputSameDT=on  OutDataTypeStr=Inherit: Same as first input
  k x j : Product  SaturateOnIntegerOverflow=on  InputSameDT=on  OutDataTypeStr=Inherit: Same as first input
  Out1 : Outport
  wires:
  j x i/1 -> Mux/3
  i x k/1 -> Mux/2
  k x j/1 -> Mux/1
  Mux/1 -> Out1/1
  Demux1/1 -> j x i/2
  Demux/2 -> j x i/1
  Demux1/3 -> i x k/2
  Demux/1 -> i x k/1
  Demux1/2 -> k x j/2
  Demux/3 -> k x j/1
  B/1 -> Demux1/1
  A/1 -> Demux/1
